simulink model "Vehicle_one_DOF_0505"  (R2024a)
settings: Solver=ode4  StartTime=0.0  StopTime=2474  FixedStep=0.001  RelTol=1e-3
InitFcn:
  | Vehicle_one_DOF_motor
undefined symbols (not defined in the file or in its folder): speed_motor, torque_motor
libraries: autolibshared x5, autolibsharedcoupling x3, autolibshareddiff x1, autolibmappedmotor x1, autolibdatasheetbattery x1, slpidlib x1
(part 1 of 3)
settings Model: DataDictionary=Vehicle_one_DOF_0505.sldd  Creator=admin  LastModifiedBy=admin
settings DebuggingCC: AllowedUnitSystems=SI,English,SI (extended),CGS  AllowAutomaticUnitConversions=off

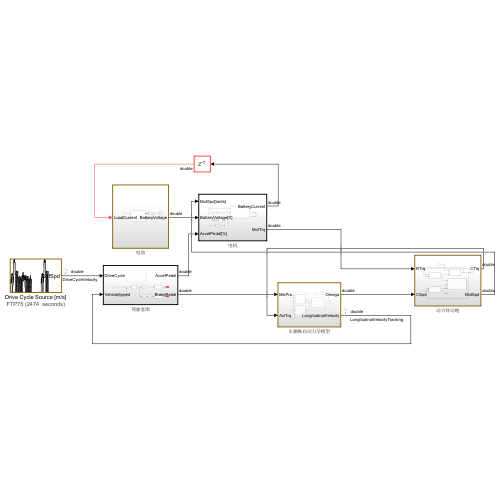
[thumbnail: Simulink's stored preview of the top-level diagram]
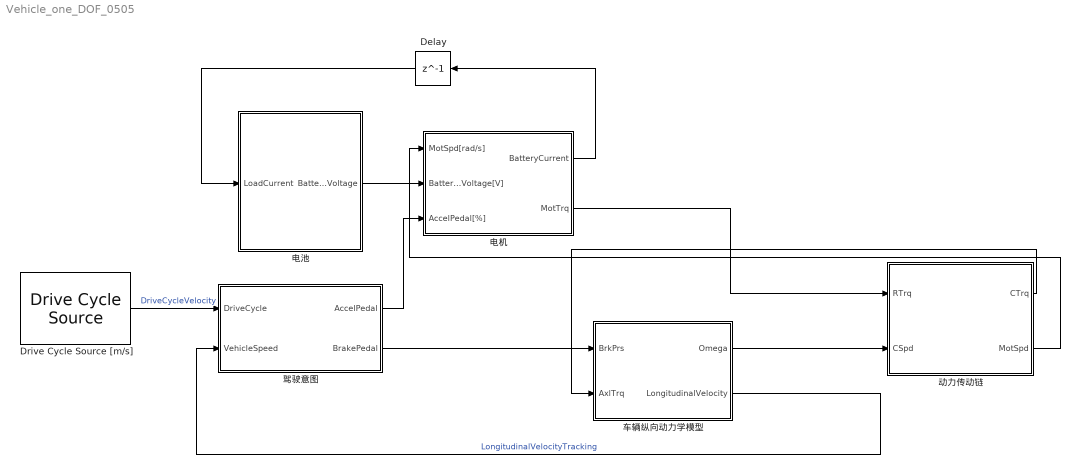
== system Vehicle_one_DOF_0505 ==
  Delay : Delay  DelayLength=1  InitialCondition=0
  Drive Cycle Source [m/s] : autolibshared/Drive Cycle Source  cycleVar=FTP75  fileVar=cycleFTP75.mat  tfinal="2474  seconds"  cycleRepeat=off  outAccPort=off  outGearPort=off  gearList=No gear data  t_wot1=5  xdot_woto=0  xdot_wot1=30  t_wot2=20  xdot_wot2=0  t_wotend=30  srcUnit=m/s  outUnit=m/s  srcAccUnit=m/s/s  outAccUnit=m/s^2  dt=0  aMode=2  faultOption=off  velBnd=2  velBndUnit=mph  inUnit=m/s  timeBnd=1  failOption=off  stopSim=off  maxFaultCnt=10  maxFaultTime=2  maxTotFaultTime=15  traceOption=off  dtTrace=1  traceWindow=10  lastDCname=FTP75  lastOutUnit=mph  lastDT=0  lastTB=1  lastSB=2  forceCalcBound=off
      settings: LibrarySourceBlock=vdynlib/Vehicle Scenarios/Drive Cycle and Maneuvers/Drive Cycle Source
  动力传动链 : Subsystem
  电机 : Subsystem
  电池 : Subsystem
  车辆纵向动力学模型 : Subsystem
  驾驶意图 : Subsystem
  wires:
  电机/2(MotTrq) -> 动力传动链/1(RTrq)
  Drive Cycle Source [m/s]/1 -> 驾驶意图/1(DriveCycle)  "DriveCycleVelocity"
  驾驶意图/2(BrakePedal) -> 车辆纵向动力学模型/1(BrkPrs)
  电池/1(BatteryVoltage) -> 电机/2(BatteryVoltage[V])
  驾驶意图/1(AccelPedal) -> 电机/3(AccelPedal[%])
  车辆纵向动力学模型/1(Omega) -> 动力传动链/2(CSpd)
  动力传动链/2(MotSpd) -> 电机/1(MotSpd[rad/s])
  动力传动链/1(CTrq) -> 车辆纵向动力学模型/2(AxlTrq)
  电机/1(BatteryCurrent) -> Delay/1
  车辆纵向动力学模型/2(LongitudinalVelocity) -> 驾驶意图/2(VehicleSpeed)  "LongitudinalVelocityTracking"
  Delay/1 -> 电池/1(LoadCurrent)

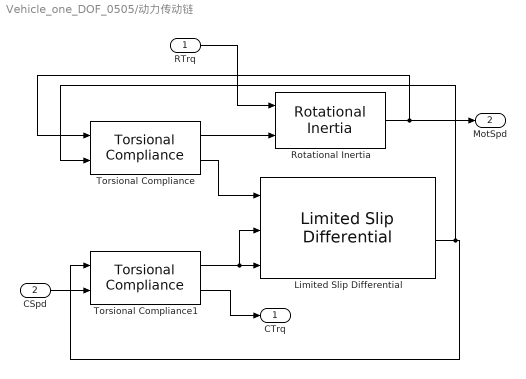
== system Vehicle_one_DOF_0505/动力传动链 ==
  RTrq : Inport
  CSpd : Inport  Port=2
  Limited Slip Differential : autolibshareddiff/Limited Slip Differential  DiffEffModelPopup=Constant  InterpMethod=Linear point-slope  extTamb=off  shaftSwitchMask=To the left of center-line  Ndiff=4  Jd=.1  bd=1e-3  Jw1=.1  bw1=1e-3  Jw2=.1  bw2=1e-3  omegaw1o=0  omegaw2o=0  eta=1  eta_tbl=reshape([0.64 0.76 0.8 0.81 0.83 0.84 0.84 0.56 0.73 0.78 0.8 0.83 0.84 0.84 0.54 0.71 0.77 0.8 0.82 0.84 0.84 0.53 0.71 0.77 0.8 0.83 0.84 0.84 0.51 0.71 0.77 0.8 0.83 0.84 0.85 0.52 0.7 0.77 0.8 0.83 0.84 0.85 0.51 0.71 0.76 0.79 0.83 0.84 0.85 0.5 0.69 0.76 0.79 0.82 0.84 0.85 0.45 0.68 0.75 0.78 0.82 0.84 0.85 0.43 0.67 0.74 0.78 0.81 0.83 0.84 0.38 0.63 0.71 0.75 0.8 0.82 0.83 0.81 0.86 0.88 0.89 0.89 0.89 0.9 0.77 0.85 0.87 0.88 0.89 0.9 0.9 0.72 0.82 0.86 0.87 0.88 0.89 0.9 0.68 0.8 0.84 0.86 0.88 0.89 0.89 0.67 0.8 0.84 0.86 0.88 0.89 0.9 0.67 0.8 0.84 0.86 0.88 0.89 0.9 0.65 0.8 0.84 0.86 0.88 0.89 0.9 0.64 0.79 0.83 0.86 0.88 0.89 0.9 0.63 0.78 0.83 0.86 0.88 0.89 0.9 0.59 0.76 0.82 0.85 0.87 0.89 0.9 0.53 0.73 0.8 0.83 0.86 0.88 0.89], 7, 11, 2)  Trq_bpts=[25, 50, 75, 100, 150, 200, 250]  omega_bpts=[52.4 78.5 105 131 157 183 209 262 314 419 524]  Temp_bpts=[290 358]  Tamb=297.15  couplingType=Pre-loaded ideal clutch  Ndisks=4  Reff=.20  Fc=500  muc=[.16 0.13 0.115 0.11 0.105 0.1025 0.10125]  dw=[0 10 20 40 60 80 100]  Tdw=[-100, -90, -50, -5, 0, 5, 50, 90, 100]  dwT=[-200, -175, -100, - 50, 0, 50, 100, 175, 200]  TTin=[-200 -175 -100 - 50 0 50 100 175 200]  Tin=[-200 -175 -100 - 50 0 50 100 175 200]  tauC=.01  IdealInterpMethod=Linear point-slope  IdealExtrapMethod=Clip  TdwInterpMethod=Linear point-slope  TdwExtrapMethod=Clip  TTinInterpMethod=Linear point-slope  TTinExtrapMethod=Clip  maxAbsSpd=5e3  aMode=2
      settings: LibrarySourceBlock=vdynlib/Powertrain/Drivetrain/Final Drive Unit/Limited Slip Differential
  Rotational Inertia : autolibsharedcoupling/Rotational Inertia  port_config=Simulink  extInfo=off  externJ=off  J=.01  b=.001  omega_o=0  blkID=0  aMode=1
      settings: LibrarySourceBlock=autolibcoupling/Rotational Inertia
  Torsional Compliance : autolibsharedcoupling/Torsional Compliance  port_config=Simulink  extInfo=off  k=5000  b=10  theta_o=0  domega_o=0  omega_c=400  blkID=0  aMode=1
  Torsional Compliance1 : autolibsharedcoupling/Torsional Compliance  port_config=Simulink  extInfo=off  k=5000  b=10  theta_o=0  domega_o=0  omega_c=400  blkID=0  aMode=1
  CTrq : Outport
  MotSpd : Outport  Port=2
  wires:
  Rotational Inertia/1 -> MotSpd/1, Torsional Compliance/1
  Torsional Compliance1/2 -> CTrq/1
  Torsional Compliance1/1 -> Limited Slip Differential/2, Limited Slip Differential/3
  CSpd/1 -> Torsional Compliance1/2
  RTrq/1 -> Rotational Inertia/1
  Limited Slip Differential/3 -> Torsional Compliance1/1, Torsional Compliance/2
  Torsional Compliance/2 -> Limited Slip Differential/1
  Torsional Compliance/1 -> Rotational Inertia/2

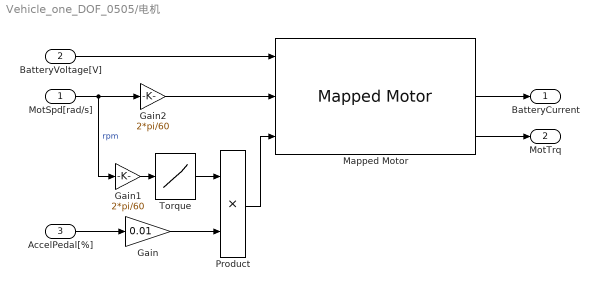
== system Vehicle_one_DOF_0505/电机 ==
  MotSpd[rad/s] : Inport
  BatteryVoltage[V] : Inport  Port=2
  AccelPedal[%] : Inport  Port=3
  Gain : Gain  Gain=0.01
  Gain1 : Gain  Gain=2*pi/60
  Gain2 : Gain  Gain=2*pi/60
  Mapped Motor : autolibmappedmotor/Mapped Motor  port_config=Speed  param_by=Tabulated torque-speed envelope  w_t=speed_motor  T_t=torque_motor  torque_max=.1  power_max=30  Tc=0.02  param_loss=Single efficiency measurement  eff=100  w_eff=375  T_eff=0.08  Piron=0  Pbase=0  w_eff_bp=[-8000 -4000 0 4000 8000]  T_eff_bp=[0 0.03 0.06 0.09]  Temp_eff_bp=[233.15 293.15 373.15]  losses_table=[1.49 1.67 2.21 3.10; 0.42 0.69 1.14 2.03; 0.06 0.24 0.78 1.68; 0.42 0.69 1.14 2.03; 1.49 1.67 2.21 3.10]  losses_table_3d=cat(3,1.05*[1.49 1.67 2.21 3.10; 0.42 0.69 1.14 2.03; 0.06 0.24 0.78 1.68; 0.42 0.69 1.14 2.03; 1.49 1.67 2.21 3.10],[1.49 1.67 2.21 3.10; 0.42 0.69 1.14 2.03; 0.06 0.24 0.78 1.68; 0.42 0.69 1.14 2.03; 1.49 1.67 2.21 3.10],1.03*[1.49 1.67 2.21 3.10; 0.42 0.69 1.14 2.03; 0.06 0.24 0.78 1.68; 0.42 0.69 1.14 2.03; 1.49 1.67 2.21 3.10])  efficiency_table=[95 95 95 95; 95 95 95 95; 95 95 95 95; 95 95 95 95; 95 95 95 95]  efficiency_table_3d=cat(3,90*ones(5,4),95*ones(5,4),92*ones(5,4))  J=5e-6  b=1e-5  omega_o=0  T_t_extended=[135.7 139.8 143.8 148.5 152.9 157.9 163.2 168.6 174 180 186.4 193.1 200 207.2 215.1 223 231.6 240.9 249.7 259.1 267.9 275 283.2 283.2 283.2 283.2 283.2 283.2 283.2 283.2 283.2 283.2 283.2 283.2 283.2 283.2 283.2 283.2 283.2 283.2 283.2 283.2 283.2 283.2 283.2 283.2 283.2 283.2 283.2 283.2 283.2 283.2 283.2 283.2 283.2 283.2 283.2 283.2 275 267.9 259.1 249.7 240.9 231.6 223 215.1 207.2 200 193.1 186.4 180 174 168.6 163.2 157.9 152.9 148.5 143.8 139.8 135.7]  w_t_extended=[-20000 -19500 -19000 -18500 -18000 -17500 -17000 -16500 -16000 -15500 -15000 -14500 -14000 -13500 -13000 -12500 -12000 -11500 -11000 -10500 -10000 -9500 -9000 -8500 -8000 -7500 -7000 -6500 -6000 -5500 -5000 -4500 -4000 -3500 -3000 -2500 -2000 -1500 -1000 -500 500 1000 1500 2000 2500 3000 3500 4000 4500 5000 5500 6000 6500 7000 7500 8000 8500 9000 9500 10000 10500 11000 11500 12000 12500 13000 13500 14000 14500 15000 15500 16000 16500 17000 17500 18000 18500 19000 19500 20000]  KLossIron=0  KLossCopper=0  x_w_eff_vec=[-8000 -4000 0 4000 8000]  x_T_eff_vec=[-0.09 -0.06 -0.03 0 0.03 0.06 0.09]  x_tmp_eff_vec=[233.15 293.15 373.15]  x_losses_mat=[3.1 2.21 1.67 1.49 1.67 2.21 3.1;2.03 1.14 0.69 0.42 0.69 1.14 2.03;1.68 0.78 0.24 0.06 0.24 0.78 1.68;2.03 1.14 0.69 0.42 0.69 1.14 2.03;3.1 2.21 1.67 1.49 1.67 2.21 3.1]  x_losses_mat_3d=cat(3,[3.255 2.3205 1.7535 1.5645 1.7535 2.3205 3.255;2.1315 1.197 0.7245 0.441 0.7245 1.197 2.1315;1.764 0.819 0.252 0.063 0.252 0.819 1.764;2.1315 1.197 0.7245 0.441 0.7245 1.197 2.1315;3.255 2.3205 1.7535 1.5645 1.7535 2.3205 3.255],[3.1 2.21 1.67 1.49 1.67 2.21 3.1;2.03 1.14 0.69 0.42 0.69 1.14 2.03;1.68 0.78 0.24 0.06 0.24 0.78 1.68;2.03 1.14 0.69 0.42 0.69 1.14 2.03;3.1 2.21 1.67 1.49 1.67 2.21 3.1],[3.193 2.2763 1.7201 1.5347 1.7201 2.2763 3.193;2.0909 1.1742 0.7107 0.4326 0.7107 1.1742 2.0909;1.7304 0.8034 0.2472 0.0618 0.2472 0.8034 1.7304;2.0909 1.1742 0.7107 0.4326 0.7107 1.1742 2.0909;3.193 2.2763 1.7201 1.5347 1.7201 2.2763 3.193])  CalLossMapData={}  CalLossWithTempMapData={}  aMode=2  RefBlkName='autolibmappedmotor/Mapped Motor'
      settings: LibrarySourceBlock=vdynlib/Powertrain/Propulsion/Mapped Motor
  Product : Product
  Torque : Lookup_n-D  NumberOfTableDimensions=1  BreakpointsForDimension1=speed_motor  Table=torque_motor  InternalRulePriority=Speed  RndMeth=Simplest
  BatteryCurrent : Outport
  MotTrq : Outport  Port=2
  wires:
  Mapped Motor/2 -> BatteryCurrent/1
  Mapped Motor/3 -> MotTrq/1
  BatteryVoltage[V]/1 -> Mapped Motor/1
  AccelPedal[%]/1 -> Gain/1
  Torque/1 -> Product/1
  Gain/1 -> Product/2
  Product/1 -> Mapped Motor/3
  MotSpd[rad/s]/1 -> Gain1/1, Gain2/1  "rpm"
  Gain1/1 -> Torque/1
  Gain2/1 -> Mapped Motor/2

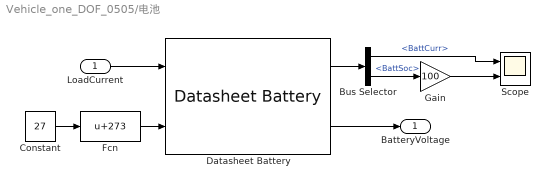
== system Vehicle_one_DOF_0505/电池 ==
  LoadCurrent : Inport
  Bus Selector : BusSelector  OutputSignals=BattCurr,BattSoc
  Constant : Constant  Value=27
  Datasheet Battery : autolibdatasheetbattery/Datasheet Battery  CapacityCtrl=Parameter  OutputVlt=Unfiltered  BattChargeMax=100  Em=[2.8 3.228 3.284 3.361 3.408 3.427 3.472 3.477 3.493 3.504 3.516 3.528 3.537 3.545 3.555 3.561 3.566 3.576 3.587 3.589 3.594 3.6 3.608 3.61 3.616 3.619 3.626 3.632 3.637 3.64 3.645 3.646 3.652 3.655 3.658 3.661 3.664 3.668 3.673 3.678 3.68 3.681 3.686 3.692 3.699 3.702 3.705 3.71 3.717 3.723 3.728 3.733 3.735 3.742 3.749 3.755 3.761 3.768 3.773 3.78 3.791 3.798 3.798 3.814 3.818 3.825 3.841 3.846 3.855 3.863 3.877 3.885 3.894 3.907 3.919 3.926 3.935 3.944 3.954 3.964 3.974 3.988 3.998 4.014 4.029 4.034 4.047 4.065 4.074 4.086 4.097 4.131 4.126 4.138 4.15 4.18 4.174 4.187 4.207 4.231 4.221]  CapLUTBp=[0 0.01 0.02 0.03 0.04 0.05 0.06 0.07 0.08 0.09 0.1 0.11 0.12 0.13 0.14 0.15 0.16 0.17 0.18 0.19 0.2 0.21 0.22 0.23 0.24 0.25 0.26 0.27 0.28 0.29 0.3 0.31 0.32 0.33 0.34 0.35 0.36 0.37 0.38 0.39 0.4 0.41 0.42 0.43 0.44 0.45 0.46 0.47 0.48 0.49 0.5 0.51 0.52 0.53 0.54 0.55 0.56 0.57 0.58 0.59 0.6 0.61 0.62 0.63 0.64 0.65 0.66 0.67 0.68 0.69 0.7 0.71 0.72 0.73 0.74 0.75 0.76 0.77 0.78 0.79 0.8 0.81 0.82 0.83 0.84 0.85 0.86 0.87 0.88 0.89 0.9 0.91 0.92 0.93 0.94 0.95 0.96 0.97 0.98 0.99 1]  RInt=[0.008846 0.009319 0.009027 0.00847 0.01032 0.01314;0.006389 0.006554 0.005553 0.005525 0.006043 0.007805;0.004364 0.004101 0.00406 0.003452 0.003846 0.004517;0.002031 0.002563 0.002532 0.00246 0.002716 0.003047;0.001443 0.001825 0.001795 0.001778 0.001924 0.002234;0.0005603 0.0007192 0.0006887 0.0007557 0.0007355 0.001014;0.001028 0.001338 0.001 0.001536 0.001546 0.002789]  BattTempBp=[243.1 253.1 263.1 273.1 283.1 298.1 313.1]  CapSOCBp=[0 0.2 0.4 0.6 0.8 1]  Ns=30  Np=2  BattCapInit=100  Tc=1/1000  Vinit=4.221  RefBlkName='autolibdatasheetbattery/Datasheet Battery'
  Fcn : Fcn  Expr=u+273
  Gain : Gain  Gain=100
  Scope : Scope  NumInputPorts=2
  BatteryVoltage : Outport
  wires:
  LoadCurrent/1 -> Datasheet Battery/1
  Datasheet Battery/2 -> BatteryVoltage/1
  Fcn/1 -> Datasheet Battery/2
  Constant/1 -> Fcn/1
  Datasheet Battery/1 -> Bus Selector/1
  Bus Selector/2 -> Gain/1  "<BattSoc>"
  Gain/1 -> Scope/2
  Bus Selector/1 -> Scope/1  "<BattCurr>"
